simulink model "MotorSubSystem"  (R2022b)
settings: Solver=VariableStepAuto  StartTime=0.0  StopTime=10.0  RelTol=1e-3
undefined symbols (not defined in the file): Kf, Kg, Kt, R
settings Model: Creator=jprmj  LastModifiedBy=jprmj

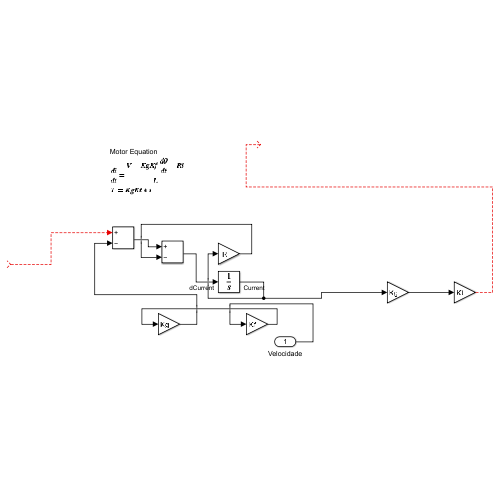
[thumbnail: Simulink's stored preview of the top-level diagram]
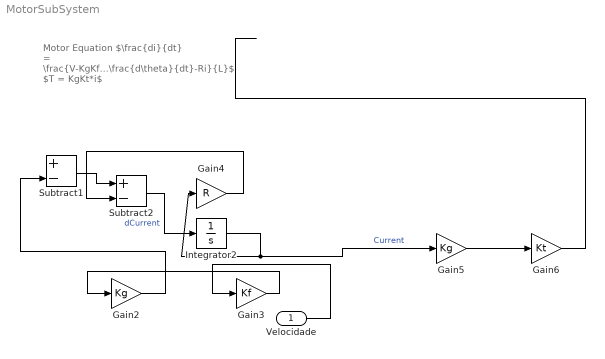
== system MotorSubSystem ==
  note: Motor Equation
      | $\frac{di}{dt} = \frac{V-KgKf\frac{d\theta}{dt}-Ri}{L}$
      | $T = KgKt*i$
  Velocidade : Inport
  Gain2 : Gain  Gain=Kg
  Gain3 : Gain  Gain=Kf
  Gain4 : Gain  Gain=R
  Gain5 : Gain  Gain=Kg
  Gain6 : Gain  Gain=Kt
  Integrator2 : Integrator
  Subtract1 : Sum  Inputs=+-
  Subtract2 : Sum  Inputs=+-
  wires:
  Gain5/1 -> Gain6/1
  Subtract2/1 -> Integrator2/1  "dCurrent"
  Velocidade/1 -> Gain3/1
  Subtract1/1 -> Subtract2/1
  Gain4/1 -> Subtract2/2
  Integrator2/1 -> Gain5/1, Gain4/1  "Current"
  Gain6/1 -> ?
  ? -> Subtract1/1
  Gain2/1 -> Subtract1/2
  Gain3/1 -> Gain2/1
